simulink library "PhD_Library"  (R2022b)
settings: Solver=VariableStepAuto  StartTime=0.0  StopTime=10.0  RelTol=1e-3
values from neighbouring files (symbols this model uses):
  Ts_control = 1/(300*Fn)    (= 5.55555555556e-05)    [Application_Script.m]    (also in ShortPulse_Script.m)
undefined symbols (not defined in the file or in its folder): D1, Delta, DiscIntNeverNeededParam, ESS, fn, Iap, PCC, Sn, tctrl, Ts_PWM, Uanp, WT
libraries: $bdroot x49, powerlib_meascontrol x35, peTransforms x28, spsSeriesRLCBranchLib x6, spsControlledVoltageSourceLib x3, spsThreePhaseVIMeasurementLib x3, spsSecondOrderFilterLib x2, spsabctodq0Lib x2, spsThreePhaseParallelRLCLoadLib x1, spsCurrentMeasurementLib x1, spsVoltageMeasurementLib x1, spsTwoLevelConverterLib x1
(part 3 of 3)

== system PhD_Library/Offshore_Oil_and_Wind/pqui_Transd_NoZeroSeq ==
  note: Akagi 1984 for p and q
      | calc. without zero seq,
      | factor 3/2 compensates for
      | amplitude invariant
      | Clarke transformation
  Vabc : Inport
  Iabc : Inport  Port=2
  Add3 : Sum  Inputs=+-
  Clarke Transform : peTransforms/Clarke Transform  PowerInvariant=off
  Clarke Transform1 : peTransforms/Clarke Transform  PowerInvariant=off
  Demux1 : Demux  Outputs=2
  Demux4 : Demux  Outputs=2
  Dot Product : DotProduct  OutDataTypeStr=Inherit: Inherit via internal rule
  Gain1 : Gain  Gain=3/2/Sn
  Gain2 : Gain  Gain=3/2/Sn
  Gain3 : Gain  Gain=1/Uanp
  Gain4 : Gain  Gain=1/Iap
  Hypot : Math  Operator=hypot  SignedPower=on  RndMeth=Zero
  Hypot1 : Math  Operator=hypot  SignedPower=on  RndMeth=Zero
  Product3 : Product
  Product4 : Product
  Selector1 : Selector  InputPortWidth=3  IndexOptions=Index vector (dialog)  Indices=[1 2]  OutputSizes=1
  Selector5 : Selector  InputPortWidth=3  IndexOptions=Index vector (dialog)  Indices=[1 2]  OutputSizes=1
  p : Outport  VectorParamsAs1DForOutWhenUnconnected=off
  q : Outport  Port=2  VectorParamsAs1DForOutWhenUnconnected=off
  v : Outport  Port=3  VectorParamsAs1DForOutWhenUnconnected=off
  i : Outport  Port=4  VectorParamsAs1DForOutWhenUnconnected=off
  wires:
  Clarke Transform1/1 -> Selector1/1
  Gain3/1 -> v/1  "v"
  Demux1/2 -> Hypot1/2, Product4/2
  Hypot1/1 -> Gain4/1  "i"
  Selector1/1 -> Demux1/1, Dot Product/2
  Selector5/1 -> Demux4/1, Dot Product/1
  Demux4/1 -> Hypot/1, Product4/1
  Hypot/1 -> Gain3/1  "v"
  Dot Product/1 -> Gain1/1  "p"
  Demux1/1 -> Hypot1/1, Product3/2
  Add3/1 -> Gain2/1  "q"
  Product4/1 -> Add3/2
  Demux4/2 -> Hypot/2, Product3/1
  Vabc/1 -> Clarke Transform/1
  Clarke Transform/1 -> Selector5/1
  Iabc/1 -> Clarke Transform1/1
  Product3/1 -> Add3/1
  Gain1/1 -> p/1  "p"
  Gain4/1 -> i/1  "i"
  Gain2/1 -> q/1  "q"

== system PhD_Library/Offshore_Oil_and_Wind/pqui_Transd_NoZeroSeq_Filter ==
  note: Akagi 1984 for p and q
      | calc. without zero seq,
      | factor 3/2 compensates for
      | amplitude invariant
      | Clarke transformation
  Vabc : Inport
  Iabc : Inport  Port=2
  Add3 : Sum  Inputs=+-
  Clarke Transform : peTransforms/Clarke Transform  PowerInvariant=off
  Clarke Transform1 : peTransforms/Clarke Transform  PowerInvariant=off
  Demux1 : Demux  Outputs=2
  Demux4 : Demux  Outputs=2
  Dot Product : DotProduct  OutDataTypeStr=Inherit: Inherit via internal rule
  Gain1 : Gain  Gain=3/2/Sn
  Gain2 : Gain  Gain=3/2/Sn
  Gain3 : Gain  Gain=1/Uanp
  Gain4 : Gain  Gain=1/Iap
  Hypot : Math  Operator=hypot  SignedPower=on  RndMeth=Zero
  Hypot1 : Math  Operator=hypot  SignedPower=on  RndMeth=Zero
  Product3 : Product
  Product4 : Product
  Rate Transition1 : RateTransition  OutPortSampleTime=Ts
  Rate Transition2 : RateTransition  OutPortSampleTime=Ts
  Second-Order Filter1 : powerlib_meascontrol/Filters/Second-Order Filter  FilterType=Lowpass  Fo=fcutoutvi  Zeta=zeta  Ts=Ts  Initialize=off  Vac_Init="[0,  0,  60]"  Vdc_Init=0  PlotResponse=off  FreqRange=[0, 1000, 0.1]
  Second-Order Filter2 : powerlib_meascontrol/Filters/Second-Order Filter  FilterType=Lowpass  Fo=fcutoutvi  Zeta=zeta  Ts=Ts  Initialize=off  Vac_Init="[0,  0,  60]"  Vdc_Init=0  PlotResponse=off  FreqRange=[0, 1000, 0.1]
  Second-Order Filter{3,5..6,8} (4 alike) : powerlib_meascontrol/Filters/Second-Order Filter  FilterType=Bandstop (Notch)  Fo=fn  Zeta=zeta  Ts=Ts  Initialize=off  Vac_Init="[0,  0,  60]"  Vdc_Init=0  PlotResponse=off  FreqRange=[0, 1000, 0.1]
  Second-Order Filter4 : powerlib_meascontrol/Filters/Second-Order Filter  FilterType=Lowpass  Fo=fcutoutpq  Zeta=zeta  Ts=Ts  Initialize=off  Vac_Init="[0,  0,  60]"  Vdc_Init=0  PlotResponse=off  FreqRange=[0, 1000, 0.1]
  Second-Order Filter7 : powerlib_meascontrol/Filters/Second-Order Filter  FilterType=Lowpass  Fo=fcutoutpq  Zeta=zeta  Ts=Ts  Initialize=off  Vac_Init="[0,  0,  60]"  Vdc_Init=0  PlotResponse=off  FreqRange=[0, 1000, 0.1]
  Selector1 : Selector  InputPortWidth=3  IndexOptions=Index vector (dialog)  Indices=[1 2]  OutputSizes=1
  Selector5 : Selector  InputPortWidth=3  IndexOptions=Index vector (dialog)  Indices=[1 2]  OutputSizes=1
  p : Outport  VectorParamsAs1DForOutWhenUnconnected=off
  q : Outport  Port=2  VectorParamsAs1DForOutWhenUnconnected=off
  v : Outport  Port=3  VectorParamsAs1DForOutWhenUnconnected=off
  i : Outport  Port=4  VectorParamsAs1DForOutWhenUnconnected=off
  wires:
  Clarke Transform1/1 -> Selector1/1
  Gain3/1 -> Second-Order Filter2/1  "v"
  Demux1/2 -> Hypot1/2, Product4/2
  Hypot1/1 -> Gain4/1  "i"
  Selector1/1 -> Demux1/1, Dot Product/2
  Selector5/1 -> Demux4/1, Dot Product/1
  Demux4/1 -> Hypot/1, Product4/1
  Hypot/1 -> Gain3/1  "v"
  Iabc/1 -> Rate Transition2/1
  Dot Product/1 -> Gain1/1  "p"
  Demux1/1 -> Hypot1/1, Product3/2
  Add3/1 -> Gain2/1  "q"
  Vabc/1 -> Rate Transition1/1
  Product4/1 -> Add3/2
  Demux4/2 -> Hypot/2, Product3/1
  Rate Transition1/1 -> Clarke Transform/1
  Clarke Transform/1 -> Selector5/1
  Rate Transition2/1 -> Clarke Transform1/1
  Product3/1 -> Add3/1
  Gain1/1 -> Second-Order Filter7/1  "p"
  Gain4/1 -> Second-Order Filter1/1  "i"
  Gain2/1 -> Second-Order Filter4/1  "q"
  Second-Order Filter2/1 -> Second-Order Filter5/1
  Second-Order Filter5/1 -> v/1
  Second-Order Filter1/1 -> Second-Order Filter3/1
  Second-Order Filter3/1 -> i/1
  Second-Order Filter4/1 -> Second-Order Filter6/1
  Second-Order Filter6/1 -> q/1
  Second-Order Filter8/1 -> p/1
  Second-Order Filter7/1 -> Second-Order Filter8/1

== system PhD_Library/Offshore_Oil_and_Wind/LSC_LCL_Trafo/INV_DClink ==
  CM : spsCurrentMeasurementLib/Current Measurement  PhasorSimulation=off  OutputType=Complex  PSBequivalent=0
  VM1 : spsVoltageMeasurementLib/Voltage Measurement  PhasorSimulation=off  OutputType=Complex  PSBequivalent=0
  Pin : PMIOPort  Side=Left
  Min : PMIOPort  Port=2  Side=Left
  Pout : PMIOPort  Port=3  Side=Right
  Mout : PMIOPort  Port=4  Side=Right
  Vdc : Outport  VectorParamsAs1DForOutWhenUnconnected=off
  Idc : Outport  Port=2  VectorParamsAs1DForOutWhenUnconnected=off
  wires:
  CM/1 -> Idc/1
  VM1/1 -> Vdc/1
  connections:
  VM1/LConn2 -- Mout/RConn1 -- Min/RConn1
  VM1/LConn1 -- CM/LConn1 -- Pin/RConn1
  CM/RConn1 -- Pout/RConn1

== matlab function PhD_Library/Adaptive Moving Averages/AMA with insertion pointer driven buffer/MATLAB Function ==
  data: x input; xavg output; n input; Nb input; xacc output; xdec output
%%%%%%%%%%%%%%%%%%%%%%%%%%%%%%%%%%%%%%%%%%%%%%%%%%%%%%%%%%%%%%%%%%%%%%%%%%
% Adaptive Moving Average Block
%%%%%%%%%%%%%%%%%%%%%%%%%%%%%%%%%%%%%%%%%%%%%%%%%%%%%%%%%%%%%%%%%%%%%%%%%%
function [xavg, xacc, xdec]  = AMAInsertionPntrDriven( x, n, Nb)

persistent buffer bufferlen rzero izero rone ione Nb_fix xavg_internal nold
 
for_acc_internal = 0;
for_dec_internal = 0;

%%%%%%%%%%%%%%%%%%%%%%%%%%%%%%%%%%
% Values of at the first cycle
%%%%%%%%%%%%%%%%%%%%%%%%%%%%%%%%%%
if isempty(buffer)
    %Nb should be larger than 2
    if Nb < 1
        %lenght of the buffer is Nb+1
        Nb_fix = 1;
        bufferlen = 2;
    else
        Nb_fix = round(Nb); %lenght of the buffer is Nb+1
        bufferlen = Nb_fix + 1;
    end
    
    %create the buffer with zeros 
    buffer = zeros(bufferlen,1);
    
    %check is n smaller or equal to Nb
    if n > Nb_fix
        n = Nb_fix;
    else
        if n < 1
            n = 1; 
        else
            n = round(n);
        end
    end
    
    %initialize pointers
    rzero = 0;
    izero = rzero + n;
    
    rone = rzero + 1;
    ione = izero + 1;
    
    %first insertion 
    %bufferlen = Nb+1 so I can write to the buffer first
    buffer(ione) = x/n;
    
    %calculating value for accumulation
    for_acc_internal = x/n;
    for_dec_internal = 0;
    
    %accumulator
    xavg_internal = for_acc_internal; 
    nold = n;
else
%%%%%%%%%%%%%%%%%%%%%%%%%%%%%%%%%%
% Here the function starts actually
%%%%%%%%%%%%%%%%%%%%%%%%%%%%%%%%%%
    %check if n smaller or equal to Nb
    if n > Nb_fix
        n = Nb_fix;
    else
        if n < 1
            n = 1; 
        else
            n = round(n);
        end
    end
    
    %insertion pointer moves forward, slot is replaced
    %bufferlen = Nb+1 so I can write to the buffer first
    izero = round( mod(izero + 1, bufferlen));
    ione = izero + 1;
    buffer(ione) = x/n;
    for_acc_internal = x/n; 
    
    %retrieval logic
    if n >= nold
        %retrieval pointer can jump backwards (as I had zeroed the buffer
        %after retrievals)
        rzero = round( mod(izero - n, bufferlen));
        rone = rzero + 1;
        for_dec_internal = buffer(rone);
        buffer(rone) = 0;
        nold = n;
    else
        jump = nold - n;
        for aux=0:jump
            rzero = round( mod(rzero + 1, bufferlen));
            rone = rzero + 1;
            for_dec_internal = for_dec_internal + buffer(rone);
            buffer(rone) = 0;
            nold = n;
        end
    end
    
    %accumulation
    xavg_internal = xavg_internal + for_acc_internal - for_dec_internal; 
end

xacc = for_acc_internal;
xdec = for_dec_internal;
xavg = xavg_internal;

== matlab function PhD_Library/Adaptive Moving Averages/AMA with retrieval pointer driven buffer/MATLAB Function ==
  data: x input; xavg output; n input; Nb input; xacc output; xdec output
%%%%%%%%%%%%%%%%%%%%%%%%%%%%%%%%%%%%%%%%%%%%%%%%%%%%%%%%%%%%%%%%%%%%%%%%%%
% Adaptive Moving Average Block
%%%%%%%%%%%%%%%%%%%%%%%%%%%%%%%%%%%%%%%%%%%%%%%%%%%%%%%%%%%%%%%%%%%%%%%%%%
% Prog/rev history
%   Mota - 2020-11-24: first release
function [xavg, xacc, xdec]  = AMARetrievalPntrDriven( x, n, Nb)

persistent buffer bufferlen r i Nb_fix xavg_internal

for_acc_internal = 0;
for_dec_internal = 0;

%%%%%%%%%%%%%%%%%%%%%%%%%%%%%%%%%%
% Values at the first cycle
%%%%%%%%%%%%%%%%%%%%%%%%%%%%%%%%%%
if isempty(buffer)
    %Nb should be larger than 1
    if Nb < 1
        %lenght of the buffer is Nb+1
        Nb_fix = 1;
        bufferlen = 2;
    else
        Nb_fix = round(Nb); %lenght of the buffer is Nb+1
        bufferlen = Nb_fix + 1;
    end
    
    %create the buffer with zeros 
    buffer = zeros(bufferlen,1);
    
    %check is n smaller or equal to Nb
    if n > Nb_fix
        n = Nb_fix;
    else
        if n < 1
            n = 1; 
        else
            n = round(n);
        end
    end
    
    %initialize pointers
    r = 1;
    i = r + n;
    
    %first sum 
    buffer(i) = buffer(i) + x/n;
    
    %calculating value for accumulation
    for_acc_internal = x/n;
    for_dec_internal = 0;
    
    %accumulator
    %xavg_internal = for_acc_internal - for_dec_internal; %first cycle, for_dec_internal=0
    xavg_internal = for_acc_internal; 
else
%%%%%%%%%%%%%%%%%%%%%%%%%%%%%%%%%%
% Here the function starts actually
%%%%%%%%%%%%%%%%%%%%%%%%%%%%%%%%%%
    %check if n smaller or equal to Nb
    if n > Nb_fix
        n = Nb_fix;
    else
        if n < 1
            n = 1; 
        else
            n = round(n);
        end
    end
    
    %pointer update
    r = r + 1;
    r = round( mod(r - 1, bufferlen) + 1); %mod works with index starting at zero, but matlab works with index on 1 
    i = round( mod(r - 1 + n, bufferlen) + 1);
    
    %insertion (sum)
    for_acc_internal = x/n; 
    buffer(i) = buffer(i) + for_acc_internal;
        
    %retrieval and zeroing 
    for_dec_internal = buffer(r);
    buffer(r) = 0; 
    
    %accumulation
    xavg_internal = xavg_internal + for_acc_internal - for_dec_internal; 
end

xacc = for_acc_internal;
xdec = for_dec_internal;
xavg = xavg_internal;

== matlab function PhD_Library/Adaptive Moving Averages/Subsystem/MATLAB Function ==
  data: x input; xavg output; xavground output; n input; Nb input; xavgceil output; xavgfloor output; xavgweigthed output; nr output; nf output; nc output; changecnt output
%%%%%%%%%%%%%%%%%%%%%%%%%%%%%%%%%%%%%%%%%%%%%%%%%%%%%%%%%%%%%%%%%%%%%%%%%%
% Adaptive Moving Average Block
%%%%%%%%%%%%%%%%%%%%%%%%%%%%%%%%%%%%%%%%%%%%%%%%%%%%%%%%%%%%%%%%%%%%%%%%%%
% Prog/rev history
%   Mota - 2020-12-08: first release

function [xavg, xavground, xavgceil, xavgfloor, xavgweigthed, nr, nf, nc, changecnt]  = AMARetrievalPntrDriven( x, n, Nb)

persistent bufferlen Nb_fix
persistent bufferround nround rround iround
persistent bufferceil nceil rceil iceil
persistent bufferfloor nfloor rfloor ifloor
persistent xavg_internal_ceil xavg_internal_round xavg_internal_floor
persistent old_nceil k_change_counter

for_acc_internal_ceil = 0;
for_dec_internal_ceil = 0;

for_acc_internal_round = 0;
for_dec_internal_round = 0;

for_acc_internal_floor = 0;
for_dec_internal_floor = 0;

nnow = n; 

%%%%%%%%%%%%%%%%%%%%%%%%%%%%%%%%%%
% Values of at the first cycle
%%%%%%%%%%%%%%%%%%%%%%%%%%%%%%%%%%
if isempty(bufferceil)
    %Nb should be larger than 1
    if Nb < 1
        %lenght of the buffer is Nb+1
        Nb_fix = 1;
        bufferlen = 2;
    else
        Nb_fix = round(Nb);%lenght of the buffer is Nb+1
        bufferlen = round(Nb_fix+1);
    end
    
    %initialize the buffer
    bufferceil = zeros(bufferlen,1);
    bufferround = zeros(bufferlen,1);
    bufferfloor = zeros(bufferlen,1);
    
    %check is n smaller or equal to Nb
    if nnow > Nb_fix
        nnow = Nb_fix;
        nceil = Nb_fix;
        nround = Nb_fix;
        nfloor = Nb_fix;
    else
        if nnow < 1
            nnow = 1;
            nceil = 1;
            nround = 1;
            nfloor = 1;
        else
            nceil = ceil(nnow);
            nround = round(nnow);
            nfloor = floor(nnow);
        end
    end
    
    %detecting change in ceiling
    old_nceil = nceil;
    k_change_counter = 0; 
    
    %initialize pointers
    rceil = 1;
    iceil = rceil + nceil;
    
    rround = 1;
    iround = rround + nround;
        
    rfloor = 1;
    ifloor = rfloor + nfloor;
        
    %first sum 
    bufferceil(iceil) = bufferceil(iceil) + x/nceil;
    bufferround(iround) = bufferround(iround) + x/nround;
    bufferfloor(ifloor) = bufferfloor(ifloor) + x/nfloor;
    
    %calculating value for accumulation
    for_acc_internal_ceil  = x/nceil;
    for_dec_internal_ceil = 0;
    
    for_acc_internal_round  = x/nround;
    for_dec_internal_round = 0;        
    
    for_acc_internal_floor  = x/nfloor;
    for_dec_internal_floor = 0;
        
    %accumulator
    xavg_internal_ceil = for_acc_internal_ceil; 
    xavg_internal_round = for_acc_internal_round; 
    xavg_internal_floor = for_acc_internal_floor; 
else
%%%%%%%%%%%%%%%%%%%%%%%%%%%%%%%%%%
% Here the function starts actually
%%%%%%%%%%%%%%%%%%%%%%%%%%%%%%%%%%
    %check is n smaller or equal to Nb
    if nnow > Nb_fix
        nnow = Nb_fix;
        nceil = Nb_fix;
        nround = Nb_fix;
        nfloor = Nb_fix;
    else
        if nnow < 1
            nnow = 1;
            nceil = 1;
            nround = 1;
            nfloor = 1;
        else
            nceil = ceil(nnow);
            nround = round(nnow);
            nfloor = floor(nnow);
        end
    end
    
    %pointer update
    %mod works from zero, matlab arrays start at index 1
    rceil = rceil + 1;
    rceil = round( mod(rceil - 1, bufferlen)+1); 
    iceil = round( mod(rceil - 1 + nceil, bufferlen) + 1);

    rround = rround + 1;
    rround = round( mod(rround - 1, bufferlen)+1); 
    iround = round( mod(rround - 1 + nround, bufferlen) + 1);
    
    rfloor = rfloor + 1;
    rfloor = round( mod(rfloor - 1, bufferlen)+1); 
    ifloor = round( mod(rfloor - 1 + nfloor, bufferlen) + 1);

    %insertion (sum)
    for_acc_internal_ceil = x/nceil; 
    bufferceil(iceil) = bufferceil(iceil) + for_acc_internal_ceil;

    for_acc_internal_round = x/nround; 
    bufferround(iround) = bufferround(iround) + for_acc_internal_round;
    
    for_acc_internal_floor = x/nfloor; 
    bufferfloor(ifloor) = bufferfloor(ifloor) + for_acc_internal_floor;

    
    %retrieval and zeroing 
    for_dec_internal_ceil = bufferceil(rceil);
    bufferceil(rceil) = 0; 

    for_dec_internal_round = bufferround(rround);
    bufferround(rround) = 0; 
        
    for_dec_internal_floor = bufferfloor(rfloor);
    bufferfloor(rfloor) = 0; 
    
    
    %accumulation
    xavg_internal_ceil = xavg_internal_ceil + for_acc_internal_ceil - for_dec_internal_ceil; 
    xavg_internal_round = xavg_internal_round + for_acc_internal_round - for_dec_internal_round; 
    xavg_internal_floor = xavg_internal_floor + for_acc_internal_floor - for_dec_internal_floor; 
end

xavgceil = xavg_internal_ceil;
xavground = xavg_internal_round;
xavgfloor = xavg_internal_floor;
xavgweigthed = (nnow - nfloor) * xavg_internal_ceil + (1 - nnow + nfloor) * xavg_internal_floor;
%alpha = (nnow - nfloor);
%oneminusalpha = (1 - nnow + nfloor);

nr = nround;
nf = nfloor;
nc = nceil;
changenc = 0;

%Check for changes in nceil and start a timer
if old_nceil ~= nceil
    changenc = 1;
    k_change_counter = 1; 
else
    if k_change_counter > 0
        k_change_counter = k_change_counter  + 1;
        if k_change_counter > nceil
            changenc = 0; 
            k_change_counter = 0;
        else
            changenc = 1;
        end
    end
end

if changenc == 1
    xavg = xavg_internal_round;
else
    xavg = (nnow - nfloor) * xavg_internal_ceil + (1 - nnow + nfloor) * xavg_internal_floor;
end
old_nceil = nceil;
changecnt = k_change_counter;
